simulink model "dcdc_buck_dual_loop_switching"  (R2024b)
settings: Solver=ode4  StartTime=0.0  StopTime=0.04  FixedStep=1e-06  RelTol=1e-3
model workspace (MAT data in the model file):
  Ki_i = 900
  Ki_v = 110
  Kp_i = 0.07
  Kp_v = 0.2
settings Model: Creator=XingTong  LastModifiedBy=XingTong

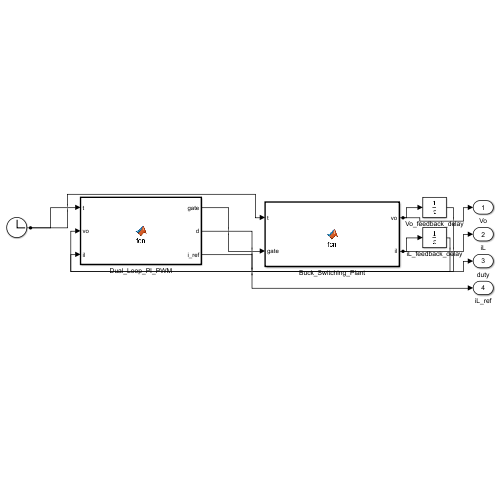
[thumbnail: Simulink's stored preview of the top-level diagram]
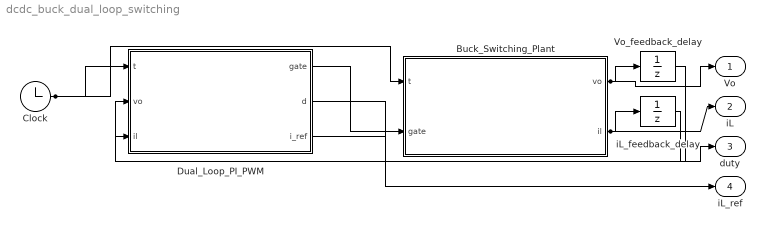
== system dcdc_buck_dual_loop_switching ==
  Buck_Switching_Plant : MATLAB Function  TreatAsAtomicUnit=on
  Clock : Clock
  Dual_Loop_PI_PWM : MATLAB Function  TreatAsAtomicUnit=on
  Vo_feedback_delay : UnitDelay  SampleTime=1e-06  HasFrameUpgradeWarning=on
  iL_feedback_delay : UnitDelay  SampleTime=1e-06  HasFrameUpgradeWarning=on
  Vo : Outport
  iL : Outport  Port=2
  duty : Outport  Port=3
  iL_ref : Outport  Port=4
  wires:
  Clock/1 -> Dual_Loop_PI_PWM/1(t), Buck_Switching_Plant/1(t)
  Buck_Switching_Plant/1(vo) -> Vo_feedback_delay/1, Vo/1
  Buck_Switching_Plant/2(il) -> iL_feedback_delay/1, iL/1
  Vo_feedback_delay/1 -> Dual_Loop_PI_PWM/2(vo)
  iL_feedback_delay/1 -> Dual_Loop_PI_PWM/3(il)
  Dual_Loop_PI_PWM/1(gate) -> Buck_Switching_Plant/2(gate)
  Dual_Loop_PI_PWM/2(d) -> duty/1
  Dual_Loop_PI_PWM/3(i_ref) -> iL_ref/1

== matlab function dcdc_buck_dual_loop_switching/Buck_Switching_Plant ==
  data: t input; vo output; gate input; il output
function [vo,il] = fcn(t,gate)
persistent x_vo x_il
vo = 0; il = 0;
if isempty(x_vo)
    x_vo = 0; x_il = 0;
end
Ts = 9.9999999999999995e-07; L = 0.00022000000000000001; C = 0.00046999999999999999; Vd = 0.69999999999999996;
Vin = 48;
R = 4.7999999999999998;
if t >= 0.021999999999999999
    R = R * 0.5;
end
if t >= 0.029999999999999999
    Vin = Vin * 0.90000000000000002;
end
if gate > 0.5
    vL = Vin - x_vo;
else
    vL = -Vd - x_vo;
end
x_il = max(0, x_il + Ts * vL / L);
x_vo = max(0, x_vo + Ts * (x_il - x_vo/R) / C);
vo = x_vo; il = x_il;
end

== matlab function dcdc_buck_dual_loop_switching/Dual_Loop_PI_PWM ==
  data: t input; gate output; vo input; il input; d output; i_ref output
function [gate,d,i_ref] = fcn(t,vo,il)
persistent ev ei carrier
gate = 0; d = 0; i_ref = 0;
if isempty(ev)
    ev = 0; ei = 0; carrier = 0;
end
Ts = 9.9999999999999995e-07; fs = 50000;
vref = 24 * min(t/0.0080000000000000002, 1);
e_v = vref - vo;
i_unsat = 0.20000000000000001*e_v + ev;
i_ref = min(max(i_unsat, 0), 12);
if i_ref == i_unsat || sign(e_v) ~= sign(i_unsat - i_ref)
    ev = ev + 110 * e_v * Ts;
end
e_i = i_ref - il;
d_unsat = 0.070000000000000007*e_i + ei;
d = min(max(d_unsat, 0.02), 0.94999999999999996);
if d == d_unsat || sign(e_i) ~= sign(d_unsat - d)
    ei = ei + 900 * e_i * Ts;
end
carrier = carrier + fs*Ts;
if carrier >= 1
    carrier = carrier - floor(carrier);
end
gate = double(carrier < d);
end
